simulink model "Grid_SensorLayout_SpatialAllignment_Clustering"  (R2018a)
settings: Solver=FixedStepAuto  StartTime=0.0  StopTime=SimulationTime  FixedStep=SamplingTime  RelTol=1e-3
values from neighbouring files (symbols this model uses):
  ValidateGRID = true    [SensorFusion_Script0_main.m]
  ValidateLAYOUT = true    [SensorFusion_Script0_main.m]
  VisualizeCLUSTERING = true    [SensorFusion_Script0_main.m]
undefined symbols (not defined in the file or in its folder): ACTIVATE_CAM, ACTIVATE_RAD, CAM1_detTimeStamp, CAM1_MeasNoise, CAM1_objClassID, CAM1_PX, CAM1_PY, CAM1_VX, CAM1_VY, CAM2_detTimeStamp, CAM2_MeasNoise, CAM2_objClassID, CAM2_PX, CAM2_PY, CAM2_VX, CAM2_VY, CAM3_detTimeStamp, CAM3_MeasNoise, CAM3_objClassID, CAM3_PX, CAM3_PY, CAM3_VX, CAM3_VY, CAM4_detTimeStamp, CAM4_MeasNoise, CAM4_objClassID, CAM4_PX, CAM4_PY, CAM4_VX, CAM4_VY, CAM5_detTimeStamp, CAM5_MeasNoise, CAM5_objClassID, CAM5_PX, CAM5_PY, CAM5_VX, CAM5_VY, CAM6_detTimeStamp, CAM6_MeasNoise, CAM6_objClassID, CAM6_PX, CAM6_PY, CAM6_VX, CAM6_VY, CAM7_detTimeStamp, CAM7_MeasNoise, CAM7_objClassID, CAM7_PX, CAM7_PY, CAM7_VX, CAM7_VY, CAM8_detTimeStamp, CAM8_MeasNoise, CAM8_objClassID, CAM8_PX, CAM8_PY, CAM8_VX, CAM8_VY, CAM_nMeas, CAM_TYPE ... (+171)
libraries: simulink_extras x4
(part 2 of 10)

== system Grid_SensorLayout_SpatialAllignment_Clustering/OBJECT_TRACKER_SENSOR_FUSION/SENSOR_LAYOUT_AND_CHRACTERIZATION/PRE_COMPUTE_SENSOR_FOV_GRID/COMPUTE_GRID_DIMENSION ==
  note: Set_Grid_Parameters
  note: Compute_number_of_grid_cells
  note: Compute_number_of_logitudinal_Grid_Cells
  note: Compute_number_of_lateral_Grid_Cells
  Bus Creator1 : BusCreator  Inputs=3
  Bus Creator2 : BusCreator  Inputs=4
  Bus Creator3 : BusCreator  Inputs=4
  Constant1 : Constant  Value=single(1)
  Constant3 : Constant  Value=single(1)
  Data Type Conversion : DataTypeConversion  OutDataTypeStr=int32
  Data Type Conversion1 : DataTypeConversion  OutDataTypeStr=uint32
  Data Type Conversion3 : DataTypeConversion  OutDataTypeStr=int32
  Divide : Product  Inputs=*/
  Divide1 : Product  Inputs=/*
  Divide2 : Product  Inputs=*/
  Divide3 : Product  Inputs=/*
  Floor{,1..3} (4 alike) : Rounding
  Gain : Gain  Gain=single(-1)
  Gain1 : Gain  Gain=single(-1)
  GridFrontLimit : Constant  Value=xFront
  GridLeftLimit : Constant  Value=yLeft
  GridRearLimit : Constant  Value=xRear
  GridResLat : Constant  Value=yRes
  GridResLong : Constant  Value=xRes
  GridRightLimit : Constant  Value=yRight
  Minus : Sum  Inputs=+-+
  Minus1 : Sum  Inputs=+-+
  Multiply : Product
  Saturation : Saturate  UpperLimit=10  LowerLimit=0.5
  Saturation1 : Saturate  UpperLimit=10  LowerLimit=0.5
  Cx : Outport
  Cy : Outport  Port=2
  GridParam : Outport  Port=3
  wires:
  GridResLong/1 -> Saturation/1
  Saturation/1 -> [xRes], Divide1/1, Divide/2
  GridFrontLimit/1 -> [xFront], Divide/1
  Divide/1 -> Floor/1
  GridRearLimit/1 -> Gain/1
  Gain/1 -> [xRear], Divide1/2
  Divide1/1 -> Floor1/1
  Floor/1 -> Minus/1
  Floor1/1 -> Minus/2
  Constant1/1 -> Minus/3
  Divide2/1 -> Floor2/1
  GridRightLimit/1 -> [yRight], Divide2/1
  GridResLat/1 -> Saturation1/1
  Constant3/1 -> Minus1/3
  Saturation1/1 -> [yRes], Divide3/1, Divide2/2
  GridLeftLimit/1 -> Gain1/1
  Gain1/1 -> [yLeft], Divide3/2
  Floor2/1 -> Minus1/1
  Divide3/1 -> Floor3/1
  Floor3/1 -> Minus1/2
  Minus/1 -> Multiply/1, Data Type Conversion/1
  Minus1/1 -> Multiply/2, Data Type Conversion3/1
  Data Type Conversion/1 -> [nGridCellsLong]
  Multiply/1 -> Data Type Conversion1/1
  Data Type Conversion1/1 -> [nGridCells]
  [nGridCells] -> Bus Creator1/1  "nGridCells"
  [nGridCellsLat] -> Cy/1, Bus Creator2/1  "nGridCellsLat"
  [yRes] -> Bus Creator2/2  "yRes"
  [yRight] -> Bus Creator2/3  "yRight"
  [yLeft] -> Bus Creator2/4  "yLeft"
  Bus Creator2/1 -> Bus Creator1/3  "yGridParameters"
  Data Type Conversion3/1 -> [nGridCellsLat]
  [nGridCellsLong] -> Cx/1, Bus Creator3/1  "nGridCellsLong"
  [xRear] -> Bus Creator3/4  "xRear"
  Bus Creator3/1 -> Bus Creator1/2  "xGridParameters"
  [xRes] -> Bus Creator3/2  "xRes"
  [xFront] -> Bus Creator3/3  "xFront"
  Bus Creator1/1 -> GridParam/1

== system Grid_SensorLayout_SpatialAllignment_Clustering/OBJECT_TRACKER_SENSOR_FUSION/SENSOR_LAYOUT_AND_CHRACTERIZATION/PRE_COMPUTE_SENSOR_FOV_GRID/COMPUTE_RADAR_SNSR_GRID ==
  SnsrParam : Inport
  GridParam : Inport  Port=2
  GridIDVector : Inport  Port=3
  ComputeCoverageANDConfidence : Subsystem  TreatAsAtomicUnit=on
  GET_SENSOR_PARAMETERS : Subsystem
  SENSOR_LOOP : ForIterator  ResetStates=reset  IterationLimit=nRadars  IterationVariableDataType=int8
  Unit Delay : UnitDelay  InitialCondition=RegionConfidenceRAD  SampleTime=-1
  Unit Delay1 : UnitDelay  InitialCondition=FOVOverlapRAD  SampleTime=-1
  Width : Width
  RegionConfidence : Outport
  FOVOverlap : Outport  Port=2
  wires:
  GridIDVector/1 -> ComputeCoverageANDConfidence/3(GridIDVector), Width/1
  Width/1 -> ComputeCoverageANDConfidence/2(nGridCells)
  SENSOR_LOOP/1 -> ComputeCoverageANDConfidence/5(SensorID), GET_SENSOR_PARAMETERS/1(SensorID)
  SnsrParam/1 -> GET_SENSOR_PARAMETERS/2(SensorParam)
  GET_SENSOR_PARAMETERS/1(extrinsic) -> ComputeCoverageANDConfidence/6(SensorExtrinsic)
  GET_SENSOR_PARAMETERS/2(intrinsic) -> ComputeCoverageANDConfidence/7(SensorIntrinsic)
  GridParam/1 -> ComputeCoverageANDConfidence/4(GridParam)
  ComputeCoverageANDConfidence/1(RegionConfidence) -> Unit Delay/1, RegionConfidence/1
  ComputeCoverageANDConfidence/2(FOVOverlap) -> Unit Delay1/1, FOVOverlap/1
  Unit Delay/1 -> ComputeCoverageANDConfidence/1(RegionConfidenceArray)
  Unit Delay1/1 -> ComputeCoverageANDConfidence/8(FOVOverlapArray)

== system Grid_SensorLayout_SpatialAllignment_Clustering/OBJECT_TRACKER_SENSOR_FUSION/SENSOR_LAYOUT_AND_CHRACTERIZATION/PRE_COMPUTE_SENSOR_FOV_GRID/CREATE_GRID ==
  Cx : Inport
  Cy : Inport  Port=2
  GridParam : Inport  Port=3
  For Iterator : ForIterator  ResetStates=reset  IterationSource=external
  For Iterator Subsystem : Subsystem  TreatAsAtomicUnit=on
  Unit Delay : UnitDelay  InitialCondition=GridCellIDs  SampleTime=-1
  CellIDVectorUpd : Outport
  wires:
  For Iterator/1 -> For Iterator Subsystem/1(xIndex)
  GridParam/1 -> For Iterator Subsystem/3(GridParam)
  Cx/1 -> For Iterator/1
  Cy/1 -> For Iterator Subsystem/2(Cy)
  For Iterator Subsystem/1(CellIDVectorUpd) -> Unit Delay/1, CellIDVectorUpd/1
  Unit Delay/1 -> For Iterator Subsystem/4(CellIDArray)

== system Grid_SensorLayout_SpatialAllignment_Clustering/OBJECT_TRACKER_SENSOR_FUSION/SENSOR_LAYOUT_AND_CHRACTERIZATION/PRE_COMPUTE_SENSOR_FOV_GRID/SET_DATA ==
  GRID_PARAM : Inport
  RAD_REGION_CONFIDENCE : Inport  Port=2
  RAD_FOV_OVERLAP : Inport  Port=3
  CAM_REGION_CONFIDENCE : Inport  Port=4
  CAM_FOV_OVERLAP : Inport  Port=5
  Bus Creator : BusCreator  Inputs=2
  Bus Creator1 : BusCreator  Inputs=2
  Bus Creator2 : BusCreator  Inputs=3
  GRID_CHARACTERIZATION : Outport
  wires:
  Bus Creator/1 -> Bus Creator2/2  "RAD_GRID"
  CAM_REGION_CONFIDENCE/1 -> Bus Creator1/1
  CAM_FOV_OVERLAP/1 -> Bus Creator1/2
  Bus Creator1/1 -> Bus Creator2/3  "CAM_GRID"
  GRID_PARAM/1 -> Bus Creator2/1
  RAD_REGION_CONFIDENCE/1 -> Bus Creator/1
  RAD_FOV_OVERLAP/1 -> Bus Creator/2
  Bus Creator2/1 -> GRID_CHARACTERIZATION/1

== system Grid_SensorLayout_SpatialAllignment_Clustering/OBJECT_TRACKER_SENSOR_FUSION/SENSOR_LAYOUT_AND_CHRACTERIZATION/SET_SENSOR_CALLIBRATION_PARAMETER/SET_CAMERA_SENSOR_PARAM ==
  CAMSnsrParam : Inport
  GET_DATA : Subsystem
  SET_CAMERA_EXTRINSIC_PARAM : Subsystem  TreatAsAtomicUnit=on
  SET_CAMERA_INTRINSIC_PARAM : Subsystem  TreatAsAtomicUnit=on
  SET_DATA : Subsystem
  CAMSnsrParamUpd : Outport
  wires:
  SET_DATA/1(CAMSnsrParamUpd) -> CAMSnsrParamUpd/1
  CAMSnsrParam/1 -> GET_DATA/1(CAMSnsrParam)
  GET_DATA/2(CameraExtrinsics) -> SET_CAMERA_EXTRINSIC_PARAM/1(CameraCalibParam)
  GET_DATA/1(CameraIntrinsics) -> SET_CAMERA_INTRINSIC_PARAM/1(CameraCalibParam)
  SET_CAMERA_INTRINSIC_PARAM/1(CameraCalibParamSet) -> SET_DATA/1(CameraIntrinsics)
  SET_CAMERA_EXTRINSIC_PARAM/1(CameraCalibParamSet) -> SET_DATA/2(CameraExtrinsics)

== system Grid_SensorLayout_SpatialAllignment_Clustering/OBJECT_TRACKER_SENSOR_FUSION/SENSOR_LAYOUT_AND_CHRACTERIZATION/SET_SENSOR_CALLIBRATION_PARAMETER/SET_RADAR_SENSOR_PARAM ==
  RADSnsrParam : Inport
  GET_DATA : Subsystem
  SET_DATA : Subsystem
  SET_RADAR_EXTRINSIC_PARAM : Subsystem  TreatAsAtomicUnit=on
  SET_RADAR_INTRINSIC_PARAM : Subsystem  TreatAsAtomicUnit=on
  RADSnsrParamUpd : Outport
  wires:
  RADSnsrParam/1 -> GET_DATA/1(RADSnsrParam)
  SET_DATA/1(RADSnsrParamUpd) -> RADSnsrParamUpd/1
  GET_DATA/2(<RadarExtrinsics>) -> SET_RADAR_EXTRINSIC_PARAM/1(RadarCalibParam)
  SET_RADAR_EXTRINSIC_PARAM/1(RadarCalibParamSet) -> SET_DATA/2(RadarExtrinsics)  "RadarIntrinsics"
  GET_DATA/1(<RadarIntrinsics>) -> SET_RADAR_INTRINSIC_PARAM/1(RadarCalibParam)
  SET_RADAR_INTRINSIC_PARAM/1(RadarCalibParamSet) -> SET_DATA/1(RadarIntrinsics)  "RadarExtrinsics"

== system Grid_SensorLayout_SpatialAllignment_Clustering/OBJECT_TRACKER_SENSOR_FUSION/SIMPLIFIED_DBSCAN_FOR_RADAR_MEASUREMENT_GROUPING/DBSCAN_MEASUREMENT_GROUPING/CHECK_IF_CLUSTER_FORMED ==
  nPts : Inport
  Constant : Constant  Value=uint16(0)
  GreaterThan : RelationalOperator  Operator=>  OutDataTypeStr=boolean  RndMeth=Simplest
  Logical Operator : Logic  Operator=NOT  AllPortsSameDT=off  OutDataTypeStr=boolean
  NoUpd : Outport
  Upd : Outport  Port=2
  wires:
  nPts/1 -> GreaterThan/1
  GreaterThan/1 -> Logical Operator/1, Upd/1
  Constant/1 -> GreaterThan/2
  Logical Operator/1 -> NoUpd/1

== system Grid_SensorLayout_SpatialAllignment_Clustering/OBJECT_TRACKER_SENSOR_FUSION/SIMPLIFIED_DBSCAN_FOR_RADAR_MEASUREMENT_GROUPING/DBSCAN_MEASUREMENT_GROUPING/COMPUTE_MEAN_IF_CLUSTER_FORMED ==
  CLSTR_DATA : Inport
  meas : Inport  Port=2
  Enable : EnablePort
  COMPUTE_COVARIANCE : Subsystem
  COMPUTE_COVARIANCE_SUM : Subsystem  TreatAsAtomicUnit=on
  COMPUTE_MEAN : Subsystem
  COMPUTE_MEAN_SUM : Subsystem  TreatAsAtomicUnit=on
  GET_DATA : Subsystem
  CLSTR_CNTR_UPD : Outport
  CLSTR_COV_UPD : Outport  Port=2
  wires:
  GET_DATA/1(nPts) -> [nPts], COMPUTE_MEAN_SUM/2(nPoints), COMPUTE_MEAN/2(n), COMPUTE_COVARIANCE_SUM/3(nPoints)
  GET_DATA/2(<ClusterMember>) -> COMPUTE_COVARIANCE_SUM/4(ClusterMembers), [ClstrMembers]
  [Meas] -> COMPUTE_COVARIANCE_SUM/2(MeasArray)
  meas/1 -> [Meas], COMPUTE_MEAN_SUM/3(MeasArray)
  [ClstrMembers] -> COMPUTE_MEAN_SUM/1(ClusterMembers)
  COMPUTE_COVARIANCE/1(Covariance) -> CLSTR_COV_UPD/1
  [nPts] -> COMPUTE_COVARIANCE/2(n)
  COMPUTE_MEAN/1(mean) -> CLSTR_CNTR_UPD/1, COMPUTE_COVARIANCE_SUM/1(mean)
  CLSTR_DATA/1 -> GET_DATA/1(CLSTR)
  COMPUTE_MEAN_SUM/1(ClusterMeanSUM) -> COMPUTE_MEAN/1(mean_sum)
  COMPUTE_COVARIANCE_SUM/1(ClusterCovSUM) -> COMPUTE_COVARIANCE/1(covariance_sum)

== system Grid_SensorLayout_SpatialAllignment_Clustering/OBJECT_TRACKER_SENSOR_FUSION/SIMPLIFIED_DBSCAN_FOR_RADAR_MEASUREMENT_GROUPING/DBSCAN_MEASUREMENT_GROUPING/FORM_CLUSTER ==
  idx_i : Inport
  measArray : Inport  Port=2
  CLSTR_DATA : Inport  Port=3
  CHECK_CONDITION : Subsystem
  DBSCAN : Subsystem
  If : If  IfExpression=u1 ~= 0
  MERGE_SIGNALS : Subsystem
  NO_CLUSTER_FORMED : Subsystem  TreatAsAtomicUnit=on
  nPts : Outport
  isMeasVisited : Outport  Port=2
  wires:
  idx_i/1 -> DBSCAN/3(idx_i), CHECK_CONDITION/1(idx_i)
  CLSTR_DATA/1 -> CHECK_CONDITION/2(CLSTR_in)
  CHECK_CONDITION/1(isNotVisited) -> If/1
  If/1 -> DBSCAN/Action
  If/2 -> NO_CLUSTER_FORMED/Action
  measArray/1 -> DBSCAN/2(measArray)
  NO_CLUSTER_FORMED/1(CLSTR_DATA_NO_UPD) -> MERGE_SIGNALS/1(CLSTR_NO_UPD)
  NO_CLUSTER_FORMED/2(nPtsEpsNoUpd) -> MERGE_SIGNALS/2(nPtsEpsNoUpd)
  DBSCAN/1(nPtsEps) -> MERGE_SIGNALS/3(nPtsUpd)
  MERGE_SIGNALS/2(CLSTR_DATA) -> isMeasVisited/1
  CHECK_CONDITION/2(CLSTR_out) -> DBSCAN/1(CLSTR_DATA), NO_CLUSTER_FORMED/1(CLSTR_DATA)
  DBSCAN/2(CLSTR_DATA_UPD) -> MERGE_SIGNALS/4(CLSTR_UPD)
  MERGE_SIGNALS/1(nPtsEps) -> nPts/1

== system Grid_SensorLayout_SpatialAllignment_Clustering/OBJECT_TRACKER_SENSOR_FUSION/SIMPLIFIED_DBSCAN_FOR_RADAR_MEASUREMENT_GROUPING/DBSCAN_MEASUREMENT_GROUPING/IF_CLUSTER_NOT_FORMED ==
  Enable : EnablePort
  Constant : Constant  Value=single(zeros(2,1))  VectorParams1D=off
  Constant1 : Constant  Value=single(zeros(2,2))  VectorParams1D=off
  Mean : Outport
  Cov : Outport  Port=2
  wires:
  Constant/1 -> Mean/1
  Constant1/1 -> Cov/1

== system Grid_SensorLayout_SpatialAllignment_Clustering/OBJECT_TRACKER_SENSOR_FUSION/SIMPLIFIED_DBSCAN_FOR_RADAR_MEASUREMENT_GROUPING/DBSCAN_MEASUREMENT_GROUPING/MERGE_SIGNALS ==
  MeanNoUpd : Inport
  CovNoUpd : Inport  Port=2
  MeanUpd : Inport  Port=3
  CovUpd : Inport  Port=4
  CLSTR_DATA : Inport  Port=5
  Flag : Inport  Port=6
  GET_DATA_FROM_BUS : Subsystem
  SET_DATA_TO_BUS : Subsystem
  UPDATE_CLUSTER_DATA : Subsystem
  CLSTR_DATA_UPD : Outport
  wires:
  GET_DATA_FROM_BUS/1(<ClusterCenter>) -> UPDATE_CLUSTER_DATA/1(Center_ARRAY)
  GET_DATA_FROM_BUS/2(<ClusterCovariance>) -> UPDATE_CLUSTER_DATA/2(Cov_ARRAY)
  GET_DATA_FROM_BUS/3(<nClusters>) -> UPDATE_CLUSTER_DATA/3(ID)
  UPDATE_CLUSTER_DATA/1(CenterUpd) -> SET_DATA_TO_BUS/2(Mean_ARRAY)
  UPDATE_CLUSTER_DATA/2(CovUpd) -> SET_DATA_TO_BUS/3(Cov_ARRAY)
  MeanUpd/1 -> UPDATE_CLUSTER_DATA/4(mean1)
  MeanNoUpd/1 -> UPDATE_CLUSTER_DATA/5(mean2)
  CovNoUpd/1 -> UPDATE_CLUSTER_DATA/7(Cov2)
  Flag/1 -> UPDATE_CLUSTER_DATA/8(FLAG)
  CovUpd/1 -> UPDATE_CLUSTER_DATA/6(Cov1)
  CLSTR_DATA/1 -> SET_DATA_TO_BUS/1(CLSTR_DATA), GET_DATA_FROM_BUS/1(CLSTR_DATA)
  SET_DATA_TO_BUS/1("CLSTR_DATA_UPD ") -> CLSTR_DATA_UPD/1

== system Grid_SensorLayout_SpatialAllignment_Clustering/OBJECT_TRACKER_SENSOR_FUSION/SPATIAL_ALLIGNMENT/CAMERA_MEASUREMENTS_SPATIAL_ALLIGNMENT/For Iterator Subsystem ==
  CameraCallibrationParam : Inport
  RadarStartingIdx : Inport  Port=2
  C1 : Inport  Port=3
  C2 : Inport  Port=4
  C3 : Inport  Port=5
  C4 : Inport  Port=6
  C5 : Inport  Port=7
  C6 : Inport  Port=8
  C7 : Inport  Port=9
  C8 : Inport  Port=10
  For Iterator : ForIterator  ResetStates=reset  IterationLimit=nCameras
  For Iterator Subsystem : Subsystem  TreatAsAtomicUnit=on
  InformationExtraction : Subsystem
  Subsystem : Subsystem
  MaxNoValidMeas : Outport
  CameraMeasTransformed : Outport  Port=2
  CameraMeasCOVTransformed : Outport  Port=3
  CameraMeasRef : Outport  Port=4
  wires:
  CameraCallibrationParam/1 -> InformationExtraction/1(CameraCallibration)
  C1/1 -> InformationExtraction/3(C1)
  C2/1 -> InformationExtraction/4(C2)
  C3/1 -> InformationExtraction/5(C3)
  C4/1 -> InformationExtraction/6(C4)
  C5/1 -> InformationExtraction/7(C5)
  C6/1 -> InformationExtraction/8(C6)
  InformationExtraction/1(CameraCalib) -> For Iterator Subsystem/1(CameraCalibration)
  InformationExtraction/2(nCameraMeas) -> For Iterator Subsystem/2(nMeas)
  InformationExtraction/3(CameraCANBus) -> For Iterator Subsystem/3(CameraCAN)
  RadarStartingIdx/1 -> InformationExtraction/11(StartingIndexes)
  Subsystem/1(nValidMeasVector) -> MaxNoValidMeas/1
  InformationExtraction/4(MeasStartingIdx) -> Subsystem/6(StartIdx)
  C7/1 -> InformationExtraction/9(C7)
  C8/1 -> InformationExtraction/10(C8)
  For Iterator/1 -> Subsystem/1(SnsrIndex), InformationExtraction/2(CameraID)
  For Iterator Subsystem/1(nValidMeas) -> Subsystem/2(nValidMeas)
  For Iterator Subsystem/2(CameraMeasUpd) -> Subsystem/3(CameraCTSMeas)
  For Iterator Subsystem/3(CameraMeasNoiseCovUpd) -> Subsystem/4(CameraCTSNoiseCOV)
  For Iterator Subsystem/4(CameraMeasRefUpd) -> Subsystem/5(CameraCTSRef)
  Subsystem/2(CTSMat) -> CameraMeasTransformed/1
  Subsystem/4(CTSMatRef) -> CameraMeasRef/1
  Subsystem/3(CTSMatNoiseCOV) -> CameraMeasCOVTransformed/1

== system Grid_SensorLayout_SpatialAllignment_Clustering/OBJECT_TRACKER_SENSOR_FUSION/SPATIAL_ALLIGNMENT/CAMERA_MEASUREMENTS_SPATIAL_ALLIGNMENT/RadarMeasurementIndexes2 ==
  validMeasCount : Inport
  CTSmeasMAT : Inport  Port=2
  CTSCovMAT : Inport  Port=3
  CTSRefMAT : Inport  Port=4
  Add{,1..6} (7 alike) : Sum
  Assignment1 : Assignment  NumberOfDimensions=2  DiagnosticForDimensions=Warning  IndexOptions=Assign all,Starting index (dialog)  Indices=1,1  OutputSizes=1,1
  Assignment2 : Assignment  NumberOfDimensions=3  DiagnosticForDimensions=Warning  IndexOptions=Assign all,Assign all,Starting index (dialog)  Indices=1,1,1  OutputSizes=1,1,1
  Assignment3 : Assignment  NumberOfDimensions=2  DiagnosticForDimensions=Warning  IndexOptions=Assign all,Starting index (dialog)  Indices=1,1  OutputSizes=1,1
  Bus Creator1 : BusCreator  Inputs=5  OutDataTypeStr=Bus: CAM_MEAS_MAT_CTS  NonVirtualBus=on
      settings: InheritFromInputs=off
  FIND1 : Subsystem  TreatAsAtomicUnit=on
  Find Nonzero Elements1 : Find  Commented=on  NumberOfInputDimensions=3
  Mux1 : Mux  Inputs=8
  Reshape1 : Reshape  OutputDimensionality=Row vector (2-D)
  Selector : Selector  NumberOfDimensions=2  InputPortWidth=3  IndexOptions=Select all,Index vector (dialog)  Indices=1,1  OutputSizes=1,1
  Selector1 : Selector  NumberOfDimensions=2  InputPortWidth=3  IndexOptions=Select all,Index vector (dialog)  Indices=6,7  OutputSizes=1,1
  Selector11 : Selector  NumberOfDimensions=2  InputPortWidth=3  IndexOptions=Index vector (dialog),Select all  Indices=1,1  OutputSizes=1,1
  Selector12 : Selector  NumberOfDimensions=2  InputPortWidth=3  IndexOptions=Select all,Index vector (port)  Indices=1,1  OutputSizes=1,1
  Selector14 : Selector  NumberOfDimensions=2  InputPortWidth=3  IndexOptions=Select all,Index vector (port)  Indices=1,1  OutputSizes=1,1
  Selector15 : Selector  NumberOfDimensions=3  InputPortWidth=3  IndexOptions=Select all,Select all,Index vector (port)  Indices=1,1,1  OutputSizes=1,1,1
  Selector2 : Selector  NumberOfDimensions=2  InputPortWidth=3  IndexOptions=Select all,Index vector (dialog)  Indices=5,2  OutputSizes=1,1
  Selector3 : Selector  NumberOfDimensions=2  InputPortWidth=3  IndexOptions=Select all,Index vector (dialog)  Indices=5,3  OutputSizes=1,1
  Selector4 : Selector  NumberOfDimensions=2  InputPortWidth=3  IndexOptions=Select all,Index vector (dialog)  Indices=5,5  OutputSizes=1,1
  Selector5 : Selector  NumberOfDimensions=2  InputPortWidth=3  IndexOptions=Select all,Index vector (dialog)  Indices=6,6  OutputSizes=1,1
  Selector6 : Selector  NumberOfDimensions=2  InputPortWidth=3  IndexOptions=Select all,Index vector (dialog)  Indices=6,8  OutputSizes=1,1
  Selector8 : Selector  NumberOfDimensions=2  InputPortWidth=3  IndexOptions=Select all,Index vector (dialog)  Indices=5,4  OutputSizes=1,1
  CTSmeasMATout : Outport
  wires:
  validMeasCount/1 -> Selector2/1, Selector/1, Bus Creator1/4, Selector3/1, Selector6/1, Selector1/1, Selector5/1, Selector4/1, Selector8/1  "ValidMeasCountMeasCount"
  Add3/1 -> Add4/1, Mux1/5
  Selector3/1 -> Add1/2
  Add2/1 -> Add3/1, Mux1/4
  Add1/1 -> Mux1/3, Add2/1
  Selector4/1 -> Add3/2
  Selector/1 -> Mux1/1, Add/1
  Add/1 -> Add1/1, Mux1/2
  Add4/1 -> Add5/1, Mux1/6
  Selector2/1 -> Add/2
  Selector8/1 -> Add2/2
  Mux1/1 -> Reshape1/1
  Selector5/1 -> Add4/2
  Bus Creator1/1 -> CTSmeasMATout/1
  CTSRefMAT/1 -> [Ref], Selector11/1
  Selector11/1 -> FIND1/1(measIdx)
  FIND1/1(ValidIndex) -> Selector14/2, Selector12/2, Selector15/2
  CTSmeasMAT/1 -> Assignment1/1, Selector14/1
  Selector14/1 -> Assignment1/2
  Selector15/1 -> Assignment2/2
  Selector12/1 -> Assignment3/2
  CTSCovMAT/1 -> Assignment2/1, Selector15/1
  Assignment3/1 -> Bus Creator1/3  "MeasRef"
  Assignment2/1 -> Bus Creator1/2  "MeasCovariance"
  Assignment1/1 -> Bus Creator1/1  "MeasArray"
  [Ref] -> Assignment3/1, Selector12/1
  Reshape1/1 -> Bus Creator1/5  "ValidCumulativeMeasCount"
  Add5/1 -> Add6/1, Mux1/7
  Selector1/1 -> Add5/2
  Add6/1 -> Mux1/8
  Selector6/1 -> Add6/2

== system Grid_SensorLayout_SpatialAllignment_Clustering/OBJECT_TRACKER_SENSOR_FUSION/SPATIAL_ALLIGNMENT/CAMERA_MEASUREMENTS_SPATIAL_ALLIGNMENT/StartingIndexes1 ==
  SnsrCallib : Inport
  CallibrationInfoExtractor : Subsystem
  Subsystem : Subsystem
  StartingIndexes : Outport
  wires:
  CallibrationInfoExtractor/1(C1nMeas) -> Subsystem/1(C1nMeas)
  CallibrationInfoExtractor/2(C2nMeas) -> Subsystem/2(C2nMeas)
  CallibrationInfoExtractor/3(C3nMeas) -> Subsystem/3(C3nMeas)
  CallibrationInfoExtractor/4(C4nMeas) -> Subsystem/4(C4nMeas)
  CallibrationInfoExtractor/5(C5nMeas) -> Subsystem/5(C5nMeas)
  Subsystem/1(StartingIndexes) -> StartingIndexes/1
  SnsrCallib/1 -> CallibrationInfoExtractor/1(SnsrCallib)
  CallibrationInfoExtractor/6(C6nMeas) -> Subsystem/6(C6nMeas)
  CallibrationInfoExtractor/7(C7nMeas) -> Subsystem/7(C7nMeas)

== system Grid_SensorLayout_SpatialAllignment_Clustering/OBJECT_TRACKER_SENSOR_FUSION/SPATIAL_ALLIGNMENT/RADAR_MEASUREMENTS_SPATIAL_ALLIGNMENT/RADAR_MEASUREMENTS_SPATIAL_ALLIGNMENT ==
  RadarCallibrationParam : Inport
  RadarStartingIdx : Inport  Port=2
  R1 : Inport  Port=3
  R2 : Inport  Port=4
  R3 : Inport  Port=5
  R4 : Inport  Port=6
  R5 : Inport  Port=7
  R6 : Inport  Port=8
  COORDINATE_TRANSFORMATION : Subsystem  TreatAsAtomicUnit=on
  GET_DATA : Subsystem
  SENSOR_LOOP : ForIterator  ResetStates=reset  IterationLimit=nRadars
  SET_DATA : Subsystem
  RadarMeasTransformed : Outport
  RadarMeasCOVTransformed : Outport  Port=2
  RadarMeasRef : Outport  Port=3
  MaxNoValidMeas : Outport  Port=4
  wires:
  RadarCallibrationParam/1 -> GET_DATA/1(RadarCallibration)
  R1/1 -> GET_DATA/3(R1)
  R2/1 -> GET_DATA/4(R2)
  R3/1 -> GET_DATA/5(R3)
  R4/1 -> GET_DATA/6(R4)
  R5/1 -> GET_DATA/7(R5)
  R6/1 -> GET_DATA/8(R6)
  GET_DATA/1(RadarCalib) -> COORDINATE_TRANSFORMATION/1(RadarCalibration)
  GET_DATA/2(nRadarMeas) -> COORDINATE_TRANSFORMATION/2(nMeas)
  GET_DATA/3(RadarCANBus) -> COORDINATE_TRANSFORMATION/3(RadarCAN)
  RadarStartingIdx/1 -> GET_DATA/9(StartingIndexes)
  SENSOR_LOOP/1 -> SET_DATA/1(SnsrIndex), GET_DATA/2(RadarID)
  SET_DATA/1(nValidMeasVector) -> MaxNoValidMeas/1
  GET_DATA/4(MeasStartingIdx) -> SET_DATA/6(StartIdx)
  COORDINATE_TRANSFORMATION/1(nValidMeas) -> SET_DATA/2(nValidMeas)
  COORDINATE_TRANSFORMATION/2(RadarMeasUpd) -> SET_DATA/3(RadarCTSMeas)
  SET_DATA/2(CTSMat) -> RadarMeasTransformed/1
  COORDINATE_TRANSFORMATION/3(RadarMeasNoiseCovUpd) -> SET_DATA/4(RadarCTSNoiseCOV)
  COORDINATE_TRANSFORMATION/4(RadarMeasRefUpd) -> SET_DATA/5(RadarCTSRef)
  SET_DATA/4(CTSMatRef) -> RadarMeasRef/1
  SET_DATA/3(CTSMatNoiseCOV) -> RadarMeasCOVTransformed/1

== system Grid_SensorLayout_SpatialAllignment_Clustering/OBJECT_TRACKER_SENSOR_FUSION/SPATIAL_ALLIGNMENT/RADAR_MEASUREMENTS_SPATIAL_ALLIGNMENT/SET_MEASUREMENTS ==
  CTSmeasMAT : Inport
  CTSCovMAT : Inport  Port=2
  CTSRefMAT : Inport  Port=3
  validMeasCount : Inport  Port=4
  Add{,1..4} (5 alike) : Sum
  Assignment1 : Assignment  NumberOfDimensions=2  DiagnosticForDimensions=Warning  IndexOptions=Assign all,Starting index (dialog)  Indices=1,1  OutputSizes=1,1
  Assignment2 : Assignment  NumberOfDimensions=3  DiagnosticForDimensions=Warning  IndexOptions=Assign all,Assign all,Starting index (dialog)  Indices=1,1,1  OutputSizes=1,1,1
  Assignment3 : Assignment  NumberOfDimensions=2  DiagnosticForDimensions=Warning  IndexOptions=Assign all,Starting index (dialog)  Indices=1,1  OutputSizes=1,1
  Bus Creator1 : BusCreator  Inputs=5  OutDataTypeStr=Bus: RAD_MEAS_MAT_CTS  NonVirtualBus=on
      settings: InheritFromInputs=off
  FIND : Subsystem  TreatAsAtomicUnit=on
  Find Nonzero Elements1 : Find  Commented=on  NumberOfInputDimensions=3
  Mux1 : Mux  Inputs=6
  Reshape1 : Reshape  OutputDimensionality=Row vector (2-D)
  Selector : Selector  NumberOfDimensions=2  InputPortWidth=3  IndexOptions=Select all,Index vector (dialog)  Indices=1,1  OutputSizes=1,1
  Selector11 : Selector  NumberOfDimensions=2  InputPortWidth=3  IndexOptions=Index vector (dialog),Select all  Indices=1,1  OutputSizes=1,1
  Selector12 : Selector  NumberOfDimensions=2  InputPortWidth=3  IndexOptions=Select all,Index vector (port)  Indices=1,1  OutputSizes=1,1
  Selector14 : Selector  NumberOfDimensions=2  InputPortWidth=3  IndexOptions=Select all,Index vector (port)  Indices=1,1  OutputSizes=1,1
  Selector15 : Selector  NumberOfDimensions=3  InputPortWidth=3  IndexOptions=Select all,Select all,Index vector (port)  Indices=1,1,1  OutputSizes=1,1,1
  Selector2 : Selector  NumberOfDimensions=2  InputPortWidth=3  IndexOptions=Select all,Index vector (dialog)  Indices=5,2  OutputSizes=1,1
  Selector3 : Selector  NumberOfDimensions=2  InputPortWidth=3  IndexOptions=Select all,Index vector (dialog)  Indices=5,3  OutputSizes=1,1
  Selector4 : Selector  NumberOfDimensions=2  InputPortWidth=3  IndexOptions=Select all,Index vector (dialog)  Indices=5,5  OutputSizes=1,1
  Selector5 : Selector  NumberOfDimensions=2  InputPortWidth=3  IndexOptions=Select all,Index vector (dialog)  Indices=6,6  OutputSizes=1,1
  Selector8 : Selector  NumberOfDimensions=2  InputPortWidth=3  IndexOptions=Select all,Index vector (dialog)  Indices=5,4  OutputSizes=1,1
  CTSmeasMATout : Outport
  wires:
  validMeasCount/1 -> Selector2/1, Selector/1, Bus Creator1/4, Selector3/1, Selector8/1, Selector4/1, Selector5/1  "ValidMeasCountMeasCount"
  Add3/1 -> Add4/1, Mux1/5
  Selector3/1 -> Add1/2
  Add2/1 -> Add3/1, Mux1/4
  Add1/1 -> Mux1/3, Add2/1
  Selector4/1 -> Add3/2
  Selector/1 -> Mux1/1, Add/1
  Add/1 -> Add1/1, Mux1/2
  Add4/1 -> Mux1/6
  Selector2/1 -> Add/2
  Selector8/1 -> Add2/2
  Mux1/1 -> Reshape1/1
  Selector5/1 -> Add4/2
  Bus Creator1/1 -> CTSmeasMATout/1
  CTSRefMAT/1 -> [Ref], Selector11/1
  Selector11/1 -> FIND/1(measIdx)
  FIND/1(ValidIndex) -> Selector14/2, Selector12/2, Selector15/2
  CTSmeasMAT/1 -> Assignment1/1, Selector14/1
  Selector14/1 -> Assignment1/2
  Selector15/1 -> Assignment2/2
  Selector12/1 -> Assignment3/2
  CTSCovMAT/1 -> Assignment2/1, Selector15/1
  Assignment3/1 -> Bus Creator1/3  "MeasRef"
  Assignment2/1 -> Bus Creator1/2  "MeasCovariance"
  Assignment1/1 -> Bus Creator1/1  "MeasArray"
  [Ref] -> Assignment3/1, Selector12/1
  Reshape1/1 -> Bus Creator1/5  "ValidCumulativeMeasCount"

== system Grid_SensorLayout_SpatialAllignment_Clustering/OBJECT_TRACKER_SENSOR_FUSION/SPATIAL_ALLIGNMENT/RADAR_MEASUREMENTS_SPATIAL_ALLIGNMENT/StartingIndexes1 ==
  SnsrCallib : Inport
  CallibrationInfoExtractor : Subsystem
  Subsystem : Subsystem
  StartingIndexes : Outport
  wires:
  CallibrationInfoExtractor/1(R1nMeas) -> Subsystem/1(R1nMeas)
  CallibrationInfoExtractor/2(R2nMeas) -> Subsystem/2(R2nMeas)
  CallibrationInfoExtractor/3(R3nMeas) -> Subsystem/3(R3nMeas)
  CallibrationInfoExtractor/4(R4nMeas) -> Subsystem/4(R4nMeas)
  CallibrationInfoExtractor/5(R5nMeas) -> Subsystem/5(R5nMeas)
  Subsystem/1(StartingIndexes) -> StartingIndexes/1
  SnsrCallib/1 -> CallibrationInfoExtractor/1(SnsrCallib)

== system Grid_SensorLayout_SpatialAllignment_Clustering/SENSOR_MEASUREMENTS/RADAR_CAMERA_EGO_SENSOR_INTERFACE/CameraSensors/Camera1 ==
  timeIdx : Inport
  nObjCamera : Inport  Port=2
  SensorMeas : Inport  Port=3
  CHECK_IF_DATA_IS_VALID : Subsystem
  GET_DATA : Subsystem
  LOOP_OVER_CAMERAS : ForIterator  ResetStates=reset  IterationSource=external  IterationVariableDataType=int16
  SET_DATA : Subsystem
  Selector : Selector  InputPortWidth=nCameras  IndexOptions=Index vector (dialog)  Indices=1  OutputSizes=1
  C1 : Outport
  wires:
  nObjCamera/1 -> Selector/1
  LOOP_OVER_CAMERAS/1 -> [index]
  GET_DATA/5(OBJ_TYPE) -> SET_DATA/7(OBJ_TYPE)
  [px] -> SET_DATA/2(px)  "px"
  GET_DATA/7(measCaptureTime) -> SET_DATA/9(TIME_STAMP)
  SET_DATA/1(C1) -> C1/1
  [vx] -> SET_DATA/4(vx)  "vx"
  GET_DATA/1(PX) -> CHECK_IF_DATA_IS_VALID/2(px), [px]
  Selector/1 -> LOOP_OVER_CAMERAS/1
  GET_DATA/3(VX) -> CHECK_IF_DATA_IS_VALID/4(vx), [vx]
  timeIdx/1 -> GET_DATA/2(time)
  CHECK_IF_DATA_IS_VALID/1(ID) -> SET_DATA/6(id)
  SensorMeas/1 -> SET_DATA/1(SensorData)
  GET_DATA/6(NOISE_COV) -> SET_DATA/8(NOISE_COV)
  [vy] -> SET_DATA/5(vy)  "vy"
  [py] -> SET_DATA/3(py)  "py"
  GET_DATA/4(VY) -> CHECK_IF_DATA_IS_VALID/5(vy), [vy]
  GET_DATA/2(PY) -> CHECK_IF_DATA_IS_VALID/3(py), [py]
  [index] -> SET_DATA/10(iter), CHECK_IF_DATA_IS_VALID/1(idx), GET_DATA/1(idx)

== system Grid_SensorLayout_SpatialAllignment_Clustering/SENSOR_MEASUREMENTS/RADAR_CAMERA_EGO_SENSOR_INTERFACE/CameraSensors/Camera2 ==
  timeIdx : Inport
  nObjCamera : Inport  Port=2
  SensorMeas : Inport  Port=3
  ExtractMeasParam1 : Subsystem
  For Iterator : ForIterator  ResetStates=reset  IterationSource=external  IterationVariableDataType=int16
  IsValid2 : Subsystem
  Selector : Selector  InputPortWidth=nCameras  IndexOptions=Starting index (dialog)  Indices=2  OutputSizes=1
  Subsystem1 : Subsystem
  C2 : Outport
  wires:
  ExtractMeasParam1/1(PX) -> IsValid2/2(px), [px]
  ExtractMeasParam1/7(measCaptureTime) -> Subsystem1/9(TIME_STAMP)
  IsValid2/1(ID) -> Subsystem1/6(id)
  [vy] -> Subsystem1/5(vy)  "vy"
  ExtractMeasParam1/6(NOISE_COV) -> Subsystem1/8(NOISE_COV)
  [vx] -> Subsystem1/4(vx)  "vx"
  SensorMeas/1 -> Subsystem1/1(SensorData)
  nObjCamera/1 -> Selector/1
  [py] -> Subsystem1/3(py)  "py"
  For Iterator/1 -> [index]
  [index] -> Subsystem1/10(iter), IsValid2/1(idx), ExtractMeasParam1/1(idx)
  ExtractMeasParam1/4(VY) -> IsValid2/5(vy), [vy]
  [px] -> Subsystem1/2(px)  "px"
  Selector/1 -> For Iterator/1
  ExtractMeasParam1/2(PY) -> IsValid2/3(py), [py]
  Subsystem1/1(C2) -> C2/1
  ExtractMeasParam1/5(OBJ_TYPE) -> Subsystem1/7(OBJ_TYPE)
  timeIdx/1 -> ExtractMeasParam1/2(time)
  ExtractMeasParam1/3(VX) -> IsValid2/4(vx), [vx]

== system Grid_SensorLayout_SpatialAllignment_Clustering/SENSOR_MEASUREMENTS/RADAR_CAMERA_EGO_SENSOR_INTERFACE/CameraSensors/Camera3 ==
  timeIdx : Inport
  nObjCamera : Inport  Port=2
  SensorMeas : Inport  Port=3
  ExtractMeasParam1 : Subsystem
  For Iterator : ForIterator  ResetStates=reset  IterationSource=external  IterationVariableDataType=int16
  IsValid2 : Subsystem
  Selector : Selector  InputPortWidth=nCameras  IndexOptions=Starting index (dialog)  Indices=3  OutputSizes=1
  Subsystem1 : Subsystem
  C3 : Outport
  wires:
  ExtractMeasParam1/1(PX) -> IsValid2/2(px), [px]
  ExtractMeasParam1/7(measCaptureTime) -> Subsystem1/9(TIME_STAMP)
  IsValid2/1(ID) -> Subsystem1/6(id)
  [vy] -> Subsystem1/5(vy)  "vy"
  ExtractMeasParam1/6(NOISE_COV) -> Subsystem1/8(NOISE_COV)
  [vx] -> Subsystem1/4(vx)  "vx"
  SensorMeas/1 -> Subsystem1/1(SensorData)
  nObjCamera/1 -> Selector/1
  [py] -> Subsystem1/3(py)  "py"
  For Iterator/1 -> [index]
  [index] -> Subsystem1/10(iter), IsValid2/1(idx), ExtractMeasParam1/1(idx)
  ExtractMeasParam1/4(VY) -> IsValid2/5(vy), [vy]
  [px] -> Subsystem1/2(px)  "px"
  Selector/1 -> For Iterator/1
  ExtractMeasParam1/2(PY) -> IsValid2/3(py), [py]
  Subsystem1/1(C3) -> C3/1
  ExtractMeasParam1/5(OBJ_TYPE) -> Subsystem1/7(OBJ_TYPE)
  timeIdx/1 -> ExtractMeasParam1/2(time)
  ExtractMeasParam1/3(VX) -> IsValid2/4(vx), [vx]

== system Grid_SensorLayout_SpatialAllignment_Clustering/SENSOR_MEASUREMENTS/RADAR_CAMERA_EGO_SENSOR_INTERFACE/CameraSensors/Camera4 ==
  timeIdx : Inport
  nObjCamera : Inport  Port=2
  SensorMeas : Inport  Port=3
  ExtractMeasParam1 : Subsystem
  For Iterator : ForIterator  ResetStates=reset  IterationSource=external  IterationVariableDataType=int16
  IsValid2 : Subsystem
  Selector : Selector  InputPortWidth=nCameras  IndexOptions=Starting index (dialog)  Indices=4  OutputSizes=1
  Subsystem1 : Subsystem
  C4 : Outport
  wires:
  ExtractMeasParam1/1(PX) -> IsValid2/2(px), [px]
  ExtractMeasParam1/7(measCaptureTime) -> Subsystem1/9(TIME_STAMP)
  IsValid2/1(ID) -> Subsystem1/6(id)
  [vy] -> Subsystem1/5(vy)  "vy"
  ExtractMeasParam1/6(NOISE_COV) -> Subsystem1/8(NOISE_COV)
  [vx] -> Subsystem1/4(vx)  "vx"
  SensorMeas/1 -> Subsystem1/1(SensorData)
  nObjCamera/1 -> Selector/1
  [py] -> Subsystem1/3(py)  "py"
  For Iterator/1 -> [index]
  [index] -> Subsystem1/10(iter), IsValid2/1(idx), ExtractMeasParam1/1(idx)
  ExtractMeasParam1/4(VY) -> IsValid2/5(vy), [vy]
  [px] -> Subsystem1/2(px)  "px"
  Selector/1 -> For Iterator/1
  ExtractMeasParam1/2(PY) -> IsValid2/3(py), [py]
  Subsystem1/1(C4) -> C4/1
  ExtractMeasParam1/5(OBJ_TYPE) -> Subsystem1/7(OBJ_TYPE)
  timeIdx/1 -> ExtractMeasParam1/2(time)
  ExtractMeasParam1/3(VX) -> IsValid2/4(vx), [vx]

== system Grid_SensorLayout_SpatialAllignment_Clustering/SENSOR_MEASUREMENTS/RADAR_CAMERA_EGO_SENSOR_INTERFACE/CameraSensors/Camera5 ==
  timeIdx : Inport
  nObjCamera : Inport  Port=2
  SensorMeas : Inport  Port=3
  ExtractMeasParam1 : Subsystem
  For Iterator : ForIterator  ResetStates=reset  IterationSource=external  IterationVariableDataType=int16
  IsValid2 : Subsystem
  Selector : Selector  InputPortWidth=nCameras  IndexOptions=Starting index (dialog)  Indices=5  OutputSizes=1
  Subsystem1 : Subsystem
  C5 : Outport
  wires:
  ExtractMeasParam1/1(PX) -> IsValid2/2(px), [px]
  ExtractMeasParam1/7(measCaptureTime) -> Subsystem1/9(TIME_STAMP)
  IsValid2/1(ID) -> Subsystem1/6(id)
  [vy] -> Subsystem1/5(vy)  "vy"
  ExtractMeasParam1/6(NOISE_COV) -> Subsystem1/8(NOISE_COV)
  [vx] -> Subsystem1/4(vx)  "vx"
  SensorMeas/1 -> Subsystem1/1(SensorData)
  nObjCamera/1 -> Selector/1
  [py] -> Subsystem1/3(py)  "py"
  For Iterator/1 -> [index]
  [index] -> Subsystem1/10(iter), IsValid2/1(idx), ExtractMeasParam1/1(idx)
  ExtractMeasParam1/4(VY) -> IsValid2/5(vy), [vy]
  [px] -> Subsystem1/2(px)  "px"
  Selector/1 -> For Iterator/1
  ExtractMeasParam1/2(PY) -> IsValid2/3(py), [py]
  Subsystem1/1(C5) -> C5/1
  ExtractMeasParam1/5(OBJ_TYPE) -> Subsystem1/7(OBJ_TYPE)
  timeIdx/1 -> ExtractMeasParam1/2(time)
  ExtractMeasParam1/3(VX) -> IsValid2/4(vx), [vx]

== system Grid_SensorLayout_SpatialAllignment_Clustering/SENSOR_MEASUREMENTS/RADAR_CAMERA_EGO_SENSOR_INTERFACE/CameraSensors/Camera6 ==
  timeIdx : Inport
  nObjCamera : Inport  Port=2
  SensorMeas : Inport  Port=3
  ExtractMeasParam1 : Subsystem
  For Iterator : ForIterator  ResetStates=reset  IterationSource=external  IterationVariableDataType=int16
  IsValid2 : Subsystem
  Selector : Selector  InputPortWidth=nCameras  IndexOptions=Starting index (dialog)  Indices=6  OutputSizes=1
  Subsystem1 : Subsystem
  C6 : Outport
  wires:
  ExtractMeasParam1/1(PX) -> IsValid2/2(px), [px]
  ExtractMeasParam1/7(measCaptureTime) -> Subsystem1/9(TIME_STAMP)
  IsValid2/1(ID) -> Subsystem1/6(id)
  [vy] -> Subsystem1/5(vy)  "vy"
  ExtractMeasParam1/6(NOISE_COV) -> Subsystem1/8(NOISE_COV)
  [vx] -> Subsystem1/4(vx)  "vx"
  SensorMeas/1 -> Subsystem1/1(SensorData)
  nObjCamera/1 -> Selector/1
  [py] -> Subsystem1/3(py)  "py"
  For Iterator/1 -> [index]
  [index] -> Subsystem1/10(iter), IsValid2/1(idx), ExtractMeasParam1/1(idx)
  ExtractMeasParam1/4(VY) -> IsValid2/5(vy), [vy]
  [px] -> Subsystem1/2(px)  "px"
  Selector/1 -> For Iterator/1
  ExtractMeasParam1/2(PY) -> IsValid2/3(py), [py]
  Subsystem1/1(C6) -> C6/1
  ExtractMeasParam1/5(OBJ_TYPE) -> Subsystem1/7(OBJ_TYPE)
  timeIdx/1 -> ExtractMeasParam1/2(time)
  ExtractMeasParam1/3(VX) -> IsValid2/4(vx), [vx]

== system Grid_SensorLayout_SpatialAllignment_Clustering/SENSOR_MEASUREMENTS/RADAR_CAMERA_EGO_SENSOR_INTERFACE/CameraSensors/Camera7 ==
  timeIdx : Inport
  nObjCamera : Inport  Port=2
  SensorMeas : Inport  Port=3
  ExtractMeasParam1 : Subsystem
  For Iterator : ForIterator  ResetStates=reset  IterationSource=external  IterationVariableDataType=int16
  IsValid2 : Subsystem
  Selector : Selector  InputPortWidth=nCameras  IndexOptions=Starting index (dialog)  Indices=7  OutputSizes=1
  Subsystem1 : Subsystem
  C7 : Outport
  wires:
  ExtractMeasParam1/1(PX) -> IsValid2/2(px), [px]
  ExtractMeasParam1/7(measCaptureTime) -> Subsystem1/9(TIME_STAMP)
  IsValid2/1(ID) -> Subsystem1/6(id)
  [vy] -> Subsystem1/5(vy)  "vy"
  ExtractMeasParam1/6(NOISE_COV) -> Subsystem1/8(NOISE_COV)
  [vx] -> Subsystem1/4(vx)  "vx"
  SensorMeas/1 -> Subsystem1/1(SensorData)
  nObjCamera/1 -> Selector/1
  [py] -> Subsystem1/3(py)  "py"
  For Iterator/1 -> [index]
  [index] -> Subsystem1/10(iter), IsValid2/1(idx), ExtractMeasParam1/1(idx)
  ExtractMeasParam1/4(VY) -> IsValid2/5(vy), [vy]
  [px] -> Subsystem1/2(px)  "px"
  Selector/1 -> For Iterator/1
  ExtractMeasParam1/2(PY) -> IsValid2/3(py), [py]
  Subsystem1/1(C7) -> C7/1
  ExtractMeasParam1/5(OBJ_TYPE) -> Subsystem1/7(OBJ_TYPE)
  timeIdx/1 -> ExtractMeasParam1/2(time)
  ExtractMeasParam1/3(VX) -> IsValid2/4(vx), [vx]

== system Grid_SensorLayout_SpatialAllignment_Clustering/SENSOR_MEASUREMENTS/RADAR_CAMERA_EGO_SENSOR_INTERFACE/CameraSensors/Camera8 ==
  timeIdx : Inport
  nObjCamera : Inport  Port=2
  SensorMeas : Inport  Port=3
  ExtractMeasParam1 : Subsystem
  For Iterator : ForIterator  ResetStates=reset  IterationSource=external  IterationVariableDataType=int16
  IsValid2 : Subsystem
  Selector : Selector  InputPortWidth=nCameras  IndexOptions=Starting index (dialog)  Indices=8  OutputSizes=1
  Subsystem1 : Subsystem
  C8 : Outport
  wires:
  ExtractMeasParam1/1(PX) -> IsValid2/2(px), [px]
  ExtractMeasParam1/7(measCaptureTime) -> Subsystem1/9(TIME_STAMP)
  IsValid2/1(ID) -> Subsystem1/6(id)
  [vy] -> Subsystem1/5(vy)  "vy"
  ExtractMeasParam1/6(NOISE_COV) -> Subsystem1/8(NOISE_COV)
  [vx] -> Subsystem1/4(vx)  "vx"
  SensorMeas/1 -> Subsystem1/1(SensorData)
  nObjCamera/1 -> Selector/1
  [py] -> Subsystem1/3(py)  "py"
  For Iterator/1 -> [index]
  [index] -> Subsystem1/10(iter), IsValid2/1(idx), ExtractMeasParam1/1(idx)
  ExtractMeasParam1/4(VY) -> IsValid2/5(vy), [vy]
  [px] -> Subsystem1/2(px)  "px"
  Selector/1 -> For Iterator/1
  ExtractMeasParam1/2(PY) -> IsValid2/3(py), [py]
  Subsystem1/1(C8) -> C8/1
  ExtractMeasParam1/5(OBJ_TYPE) -> Subsystem1/7(OBJ_TYPE)
  timeIdx/1 -> ExtractMeasParam1/2(time)
  ExtractMeasParam1/3(VX) -> IsValid2/4(vx), [vx]

== system Grid_SensorLayout_SpatialAllignment_Clustering/SENSOR_MEASUREMENTS/RADAR_CAMERA_EGO_SENSOR_INTERFACE/EgoSensors/ExtractMeasParam ==
  timeIdx : Inport
  Constant : Constant  Value=EGO_PX
  Constant1 : Constant  Value=EGO_PY
  Constant2 : Constant  Value=EGO_VX
  Constant3 : Constant  Value=EGO_VY
  Constant4 : Constant  Value=EGO_YAW
  Constant5 : Constant  Value=EGO_YAWRATE
  Constant6 : Constant  Value=EGO_TimeStamp
  Constant7 : Constant  Value=EGO_IgnitionStatus
  EGO_IGNITION_STAT : Selector  NumberOfDimensions=2  InputPortWidth=portSize  IndexOptions=Select all,Index vector (port)  Indices=[1 3],1  OutputSizes=1,1
  EGO_PX : Selector  NumberOfDimensions=2  InputPortWidth=portSize  IndexOptions=Select all,Index vector (port)  Indices=[1 3],1  OutputSizes=1,1
  EGO_PY : Selector  NumberOfDimensions=2  InputPortWidth=portSize  IndexOptions=Select all,Index vector (port)  Indices=[1 3],1  OutputSizes=1,1
  EGO_VX : Selector  NumberOfDimensions=2  InputPortWidth=portSize  IndexOptions=Select all,Index vector (port)  Indices=[1 3],1  OutputSizes=1,1
  EGO_VY : Selector  NumberOfDimensions=2  InputPortWidth=portSize  IndexOptions=Select all,Index vector (port)  Indices=[1 3],1  OutputSizes=1,1
  EGO_YAW : Selector  NumberOfDimensions=2  InputPortWidth=portSize  IndexOptions=Select all,Index vector (port)  Indices=[1 3],1  OutputSizes=1,1
  EGO_YAWRATE : Selector  NumberOfDimensions=2  InputPortWidth=portSize  IndexOptions=Select all,Index vector (port)  Indices=[1 3],1  OutputSizes=1,1
  TIME_STAMP : Selector  NumberOfDimensions=2  InputPortWidth=portSize  IndexOptions=Select all,Index vector (port)  Indices=[1 3],1  OutputSizes=1,1
  EgoTimeStamp : Outport
  EgoPx : Outport  Port=2
  EgoPy : Outport  Port=3
  EgoVx : Outport  Port=4
  EgoVy : Outport  Port=5
  EgoYaw : Outport  Port=6
  EgoYawRate : Outport  Port=7
  EgoIgnitionStatus : Outport  Port=8
  wires:
  Constant3/1 -> EGO_VY/1
  Constant2/1 -> EGO_VX/1
  Constant/1 -> EGO_PX/1
  Constant1/1 -> EGO_PY/1
  EGO_VX/1 -> EgoVx/1
  EGO_PX/1 -> EgoPx/1
  timeIdx/1 -> EGO_PX/2, EGO_PY/2, EGO_VX/2, EGO_VY/2, EGO_YAW/2, EGO_YAWRATE/2, EGO_IGNITION_STAT/2, TIME_STAMP/2
  Constant4/1 -> EGO_YAW/1
  EGO_YAW/1 -> EgoYaw/1
  Constant6/1 -> TIME_STAMP/1
  TIME_STAMP/1 -> EgoTimeStamp/1
  EGO_YAWRATE/1 -> EgoYawRate/1
  Constant5/1 -> EGO_YAWRATE/1
  EGO_PY/1 -> EgoPy/1
  EGO_VY/1 -> EgoVy/1
  Constant7/1 -> EGO_IGNITION_STAT/1
  EGO_IGNITION_STAT/1 -> EgoIgnitionStatus/1

== system Grid_SensorLayout_SpatialAllignment_Clustering/SENSOR_MEASUREMENTS/RADAR_CAMERA_EGO_SENSOR_INTERFACE/RadarSensors/Radar1 ==
  timeIdx : Inport
  nObjRadar : Inport  Port=2
  SensorMeas : Inport  Port=3
  CHECK_IF_DATA_VALID : Subsystem
  GET_DATA : Subsystem
  LOOP_OVER_RADARS : ForIterator  ResetStates=reset  IterationSource=external  IterationVariableDataType=int16
  SET_DATA : Subsystem
  Selector : Selector  InputPortWidth=nRadars  IndexOptions=Starting index (dialog)  Indices=1  OutputSizes=1
  R1 : Outport
  wires:
  nObjRadar/1 -> Selector/1
  LOOP_OVER_RADARS/1 -> [index]
  [index] -> CHECK_IF_DATA_VALID/1(idx), GET_DATA/1(idx), SET_DATA/10(iter)
  timeIdx/1 -> GET_DATA/2(time)
  GET_DATA/1(PX) -> CHECK_IF_DATA_VALID/2(px), [px]
  GET_DATA/2(PY) -> CHECK_IF_DATA_VALID/3(py), [py]
  GET_DATA/3(VX) -> CHECK_IF_DATA_VALID/4(vx), [vx]
  GET_DATA/4(VY) -> CHECK_IF_DATA_VALID/5(vy), [vy]
  SensorMeas/1 -> SET_DATA/1(SensorData)
  [px] -> SET_DATA/2(px)  "px"
  [py] -> SET_DATA/3(py)  "py"
  [vx] -> SET_DATA/4(vx)  "vx"
  [vy] -> SET_DATA/5(vy)  "vy"
  SET_DATA/1(R1) -> R1/1
  CHECK_IF_DATA_VALID/1(ID) -> SET_DATA/6(id)
  Selector/1 -> LOOP_OVER_RADARS/1
  GET_DATA/5(SNR) -> SET_DATA/7(SNR)
  GET_DATA/6(NOISE_COV) -> SET_DATA/8(NOISE_COV)
  GET_DATA/7(measCaptureTime) -> SET_DATA/9(TIME_STAMP)

== system Grid_SensorLayout_SpatialAllignment_Clustering/SENSOR_MEASUREMENTS/RADAR_CAMERA_EGO_SENSOR_INTERFACE/RadarSensors/Radar2 ==
  timeIdx : Inport
  nObjRadar : Inport  Port=2
  SensorMeas : Inport  Port=3
  ExtractMeasParam : Subsystem
  For Iterator : ForIterator  ResetStates=reset  IterationSource=external  IterationVariableDataType=int16
  IsValid1 : Subsystem
  Selector : Selector  InputPortWidth=nRadars  IndexOptions=Starting index (dialog)  Indices=2  OutputSizes=1
  Subsystem : Subsystem
  R2 : Outport
  wires:
  [vx] -> Subsystem/4(vx)  "vx"
  Subsystem/1(R2) -> R2/1
  ExtractMeasParam/1(PX) -> IsValid1/2(px), [px]
  IsValid1/1(ID) -> Subsystem/6(id)
  [py] -> Subsystem/3(py)  "py"
  ExtractMeasParam/3(VX) -> IsValid1/4(vx), [vx]
  ExtractMeasParam/6(NOISE_COV) -> Subsystem/8(NOISE_COV)
  ExtractMeasParam/4(VY) -> IsValid1/5(vy), [vy]
  [px] -> Subsystem/2(px)  "px"
  nObjRadar/1 -> Selector/1
  SensorMeas/1 -> Subsystem/1(SensorData)
  timeIdx/1 -> ExtractMeasParam/2(time)
  [index] -> IsValid1/1(idx), ExtractMeasParam/1(idx), Subsystem/10(iter)
  [vy] -> Subsystem/5(vy)  "vy"
  ExtractMeasParam/2(PY) -> IsValid1/3(py), [py]
  For Iterator/1 -> [index]
  ExtractMeasParam/5(SNR) -> Subsystem/7(SNR)
  ExtractMeasParam/7(measCaptureTime) -> Subsystem/9(TIME_STAMP)
  Selector/1 -> For Iterator/1

== system Grid_SensorLayout_SpatialAllignment_Clustering/SENSOR_MEASUREMENTS/RADAR_CAMERA_EGO_SENSOR_INTERFACE/RadarSensors/Radar3 ==
  timeIdx : Inport
  nObjRadar : Inport  Port=2
  SensorMeas : Inport  Port=3
  ExtractMeasParam : Subsystem
  For Iterator : ForIterator  ResetStates=reset  IterationSource=external  IterationVariableDataType=int16
  IsValid1 : Subsystem
  Selector : Selector  InputPortWidth=nRadars  IndexOptions=Starting index (dialog)  Indices=3  OutputSizes=1
  Subsystem : Subsystem
  R3 : Outport
  wires:
  [vx] -> Subsystem/4(vx)  "vx"
  Subsystem/1(R3) -> R3/1
  ExtractMeasParam/1(PX) -> IsValid1/2(px), [px]
  IsValid1/1(ID) -> Subsystem/6(id)
  [py] -> Subsystem/3(py)  "py"
  ExtractMeasParam/3(VX) -> IsValid1/4(vx), [vx]
  ExtractMeasParam/6(NOISE_COV) -> Subsystem/8(NOISE_COV)
  ExtractMeasParam/4(VY) -> IsValid1/5(vy), [vy]
  [px] -> Subsystem/2(px)  "px"
  nObjRadar/1 -> Selector/1
  SensorMeas/1 -> Subsystem/1(SensorData)
  timeIdx/1 -> ExtractMeasParam/2(time)
  [index] -> IsValid1/1(idx), ExtractMeasParam/1(idx), Subsystem/10(iter)
  [vy] -> Subsystem/5(vy)  "vy"
  ExtractMeasParam/2(PY) -> IsValid1/3(py), [py]
  For Iterator/1 -> [index]
  ExtractMeasParam/5(SNR) -> Subsystem/7(SNR)
  ExtractMeasParam/7(measCaptureTime) -> Subsystem/9(TIME_STAMP)
  Selector/1 -> For Iterator/1

== system Grid_SensorLayout_SpatialAllignment_Clustering/SENSOR_MEASUREMENTS/RADAR_CAMERA_EGO_SENSOR_INTERFACE/RadarSensors/Radar4 ==
  timeIdx : Inport
  nObjRadar : Inport  Port=2
  SensorMeas : Inport  Port=3
  ExtractMeasParam : Subsystem
  For Iterator : ForIterator  ResetStates=reset  IterationSource=external  IterationVariableDataType=int16
  IsValid1 : Subsystem
  Selector : Selector  InputPortWidth=nRadars  IndexOptions=Starting index (dialog)  Indices=4  OutputSizes=1
  Subsystem : Subsystem
  R4 : Outport
  wires:
  ExtractMeasParam/2(PY) -> IsValid1/3(py), [py]
  [vy] -> Subsystem/5(vy)  "vy"
  [index] -> IsValid1/1(idx), ExtractMeasParam/1(idx), Subsystem/10(iter)
  SensorMeas/1 -> Subsystem/1(SensorData)
  ExtractMeasParam/6(NOISE_COV) -> Subsystem/8(NOISE_COV)
  ExtractMeasParam/4(VY) -> IsValid1/5(vy), [vy]
  ExtractMeasParam/3(VX) -> IsValid1/4(vx), [vx]
  timeIdx/1 -> ExtractMeasParam/2(time)
  IsValid1/1(ID) -> Subsystem/6(id)
  ExtractMeasParam/1(PX) -> IsValid1/2(px), [px]
  [vx] -> Subsystem/4(vx)  "vx"
  Selector/1 -> For Iterator/1
  nObjRadar/1 -> Selector/1
  Subsystem/1(R4) -> R4/1
  ExtractMeasParam/7(measCaptureTime) -> Subsystem/9(TIME_STAMP)
  [px] -> Subsystem/2(px)  "px"
  ExtractMeasParam/5(SNR) -> Subsystem/7(SNR)
  [py] -> Subsystem/3(py)  "py"
  For Iterator/1 -> [index]

== system Grid_SensorLayout_SpatialAllignment_Clustering/SENSOR_MEASUREMENTS/RADAR_CAMERA_EGO_SENSOR_INTERFACE/RadarSensors/Radar5 ==
  timeIdx : Inport
  nObjRadar : Inport  Port=2
  SensorMeas : Inport  Port=3
  ExtractMeasParam : Subsystem
  For Iterator : ForIterator  ResetStates=reset  IterationSource=external  IterationVariableDataType=int16
  IsValid1 : Subsystem
  Selector : Selector  InputPortWidth=nRadars  IndexOptions=Starting index (dialog)  Indices=5  OutputSizes=1
  Subsystem : Subsystem
  R5 : Outport
  wires:
  ExtractMeasParam/2(PY) -> IsValid1/3(py), [py]
  [vy] -> Subsystem/5(vy)  "vy"
  [index] -> IsValid1/1(idx), ExtractMeasParam/1(idx), Subsystem/10(iter)
  SensorMeas/1 -> Subsystem/1(SensorData)
  ExtractMeasParam/6(NOISE_COV) -> Subsystem/8(NOISE_COV)
  ExtractMeasParam/4(VY) -> IsValid1/5(vy), [vy]
  ExtractMeasParam/3(VX) -> IsValid1/4(vx), [vx]
  timeIdx/1 -> ExtractMeasParam/2(time)
  IsValid1/1(ID) -> Subsystem/6(id)
  ExtractMeasParam/1(PX) -> IsValid1/2(px), [px]
  [vx] -> Subsystem/4(vx)  "vx"
  Selector/1 -> For Iterator/1
  nObjRadar/1 -> Selector/1
  Subsystem/1(R5) -> R5/1
  ExtractMeasParam/7(measCaptureTime) -> Subsystem/9(TIME_STAMP)
  [px] -> Subsystem/2(px)  "px"
  ExtractMeasParam/5(SNR) -> Subsystem/7(SNR)
  [py] -> Subsystem/3(py)  "py"
  For Iterator/1 -> [index]

== system Grid_SensorLayout_SpatialAllignment_Clustering/SENSOR_MEASUREMENTS/RADAR_CAMERA_EGO_SENSOR_INTERFACE/RadarSensors/Radar6 ==
  timeIdx : Inport
  nObjRadar : Inport  Port=2
  SensorMeas : Inport  Port=3
  ExtractMeasParam : Subsystem
  For Iterator : ForIterator  ResetStates=reset  IterationSource=external  IterationVariableDataType=int16
  IsValid1 : Subsystem
  Selector : Selector  InputPortWidth=nRadars  IndexOptions=Starting index (dialog)  Indices=6  OutputSizes=1
  Subsystem : Subsystem
  R6 : Outport
  wires:
  ExtractMeasParam/2(PY) -> IsValid1/3(py), [py]
  [vy] -> Subsystem/5(vy)  "vy"
  [index] -> IsValid1/1(idx), ExtractMeasParam/1(idx), Subsystem/10(iter)
  SensorMeas/1 -> Subsystem/1(SensorData)
  ExtractMeasParam/6(NOISE_COV) -> Subsystem/8(NOISE_COV)
  ExtractMeasParam/4(VY) -> IsValid1/5(vy), [vy]
  ExtractMeasParam/3(VX) -> IsValid1/4(vx), [vx]
  timeIdx/1 -> ExtractMeasParam/2(time)
  IsValid1/1(ID) -> Subsystem/6(id)
  ExtractMeasParam/1(PX) -> IsValid1/2(px), [px]
  [vx] -> Subsystem/4(vx)  "vx"
  Selector/1 -> For Iterator/1
  nObjRadar/1 -> Selector/1
  Subsystem/1(R6) -> R6/1
  ExtractMeasParam/7(measCaptureTime) -> Subsystem/9(TIME_STAMP)
  [px] -> Subsystem/2(px)  "px"
  ExtractMeasParam/5(SNR) -> Subsystem/7(SNR)
  [py] -> Subsystem/3(py)  "py"
  For Iterator/1 -> [index]

== system Grid_SensorLayout_SpatialAllignment_Clustering/SENSOR_MEASUREMENTS/RADAR_CAMERA_EGO_SENSOR_INTERFACE/RoadSensors/LineSensor1 ==
  timeIdx : Inport
  nLines : Inport  Port=2
  CameraLineCoeff : Inport  Port=3
  CHECK_IF_DATA_IS_VALID : Subsystem
  GET_DATA : Subsystem
  LOOP_OVER_CAMERAS : ForIterator  ResetStates=reset  IterationSource=external  IterationVariableDataType=int16
  SET_DATA : Subsystem
  Selector : Selector  InputPortWidth=nCameras  IndexOptions=Index vector (dialog)  Indices=1  OutputSizes=1
  C1 : Outport
  wires:
  nLines/1 -> Selector/1
  LOOP_OVER_CAMERAS/1 -> [index]
  GET_DATA/5(lateralOffset) -> SET_DATA/7(lateralOffset)
  [curv] -> SET_DATA/2(curv)
  GET_DATA/9(measCaptureTime) -> SET_DATA/11(TIME_STAMP)
  SET_DATA/1(C1) -> C1/1
  [curvLen] -> SET_DATA/4(curvLen)
  GET_DATA/1(curvature) -> CHECK_IF_DATA_IS_VALID/2(curvature), [curv]
  Selector/1 -> LOOP_OVER_CAMERAS/1
  GET_DATA/3(curvLength) -> CHECK_IF_DATA_IS_VALID/4(curvLength), [curvLen]
  timeIdx/1 -> GET_DATA/2(time)
  CHECK_IF_DATA_IS_VALID/1(validID) -> SET_DATA/6(ValidID)
  CameraLineCoeff/1 -> SET_DATA/1(CameraLineCoeff)
  GET_DATA/6(xmin) -> SET_DATA/8(xmin)
  [alpha] -> SET_DATA/5(alpha)
  [curvRate] -> SET_DATA/3(curvRate)
  GET_DATA/4(headingAngle) -> CHECK_IF_DATA_IS_VALID/5(HeadingAngle), [alpha]
  GET_DATA/2(curvRate) -> CHECK_IF_DATA_IS_VALID/3(curvatureRate), [curvRate]
  [index] -> CHECK_IF_DATA_IS_VALID/1(LineID), SET_DATA/12(iter), GET_DATA/1(idx)
  GET_DATA/7(xmax) -> SET_DATA/9(xmax)
  GET_DATA/8(lineMarkWidth) -> SET_DATA/10(lineWidth)
